simulink library "IO"  (R2025a)
settings: Solver=VariableStepAuto  StartTime=0.0  StopTime=10.0  RelTol=1e-3
values from neighbouring files (symbols this model uses):
  ADCBits = 12.0    [IO.sldd]
  Vref = 5.0    [IO.sldd]
undefined symbols (not defined in the file or in its folder): Bridge, dt, H, raptor_xcp_function
libraries: Raptor_lib x133, Utilities x20, Cooling x1
(part 6 of 6)

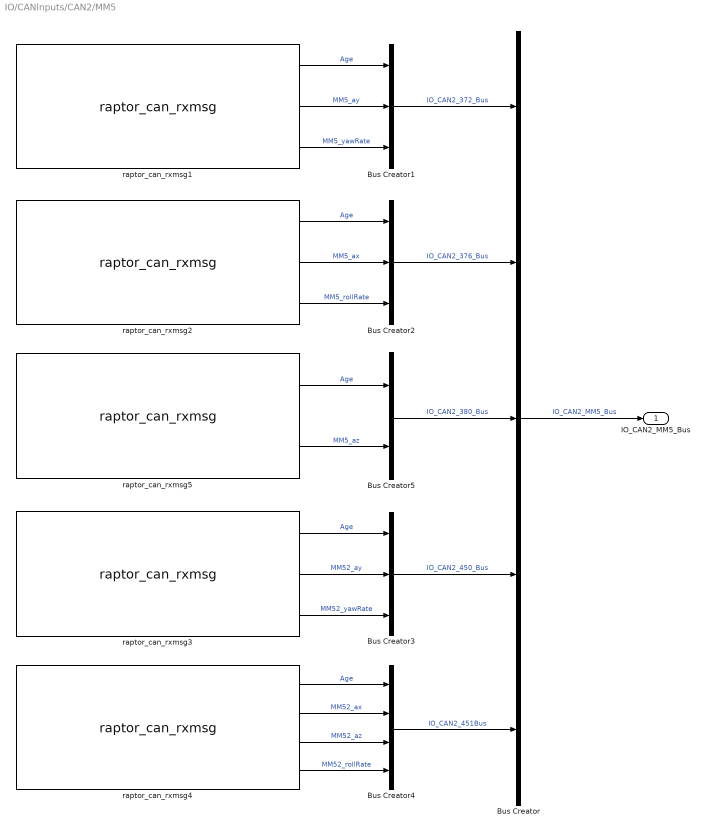
== system IO/CANInputs/CAN2/MM5 ==
  Bus Creator : BusCreator  Inputs=5
  Bus Creator1 : BusCreator  Inputs=3
  Bus Creator2 : BusCreator  Inputs=3
  Bus Creator3 : BusCreator  Inputs=3
  Bus Creator4 : BusCreator  Inputs=4
  Bus Creator5 : BusCreator  Inputs=2
  raptor_can_rxmsg1 : Raptor_lib/CAN/raptor_can_rxmsg  canDefinition=struct('dbcFile', 'SR26_CAN2.dbc','message', 'MM5_372','comment', '','signals', {{'MM5_ay','MM5_yawRate'}},'enabled', [ 1 1;],'scaled', [ 1 1;],'canBus', '''CAN2''','messageID', [ 372;],'idMask', [ 536870911;],'payloadMask', [],'payloadValue', [],'period', [ 0;],'mailbox', '''''','queueSize', [ 1;],'label', [ 0;],'ver', [ 2;],'showID', [ 0;],'showRaw', [ 0;],'showRawMsg', [ 0;],'useStartVals', [ 0;],'extendedId', [ 0;],'showAge', [ 1;],'useSimFunc', [ 0;],'sim_func_name', '''''','fill', [ 0;],'editID', [ 0;],'signalOrder', [ 1;],'signalAscDes', [ 1;],'msgLength', [ 8;])  canBus='CAN2'  mailbox=''  payloadMask=[]  payloadValue=[]  idMask=hex2dec('1FFFFFFF')  queueSize=1  showID=0  label=0  fill=0  id=372  showRaw=0  showAge=1  signalOrder=1  signalInfo={{struct('Name', 'MM5_ay','StartBit', [ 32;],'SignalSize', [ 16;],'ByteOrder', 'LittleEndian','ValueType', 'UNSIGNED','Class', 'uint16','Signed', [ 0;],'Factor', [ 0.0001274;],'Offset', [ -4.1746;],'Min', [ 0;],'Max', [ 0;],'Units', 'g','StartVal', [ 0;],'Comment', 'Acceleration Y Axis','Multiplexed', [ 0;],'Multiplexor', [ 0;],'MultiplexMode_Min', [],'MultiplexMode_Max', []),struct('Name', 'MM5_yawRate','StartBit', [ 0;],'SignalSize', [ 16;],'ByteOrder', 'LittleEndian','ValueType', 'UNSIGNED','Class', 'uint16','Signed', [ 0;],'Factor', [ 0.005;],'Offset', [ -163.9;],'Min', [ 0;],'Max', [ 0;],'Units', 'deg/sec','StartVal', [ 0;],'Comment', 'Yaw Rate','Multiplexed', [ 0;],'Multiplexor', [ 0;],'MultiplexMode_Min', [],'MultiplexMode_Max', [])}}  showRawMsg=0  useSimFunc=0  sim_func_name=''  useStartVals=0  extendedId=0
      settings: SourceProductName=Raptor
  raptor_can_rxmsg2 : Raptor_lib/CAN/raptor_can_rxmsg  canDefinition=struct('dbcFile', 'SR26_CAN2.dbc','message', 'MM5_376','comment', '','signals', {{'MM5_ax','MM5_rollRate'}},'enabled', [ 1 1;],'scaled', [ 1 1;],'canBus', '''CAN2''','messageID', [ 376;],'idMask', [ 536870911;],'payloadMask', [],'payloadValue', [],'period', [ 0;],'mailbox', '''''','queueSize', [ 1;],'label', [ 0;],'ver', [ 2;],'showID', [ 0;],'showRaw', [ 0;],'showRawMsg', [ 0;],'useStartVals', [ 0;],'extendedId', [ 0;],'showAge', [ 1;],'useSimFunc', [ 0;],'sim_func_name', '''''','fill', [ 0;],'editID', [ 0;],'signalOrder', [ 1;],'signalAscDes', [ 1;],'msgLength', [ 8;])  canBus='CAN2'  mailbox=''  payloadMask=[]  payloadValue=[]  idMask=hex2dec('1FFFFFFF')  queueSize=1  showID=0  label=0  fill=0  id=376  showRaw=0  showAge=1  signalOrder=1  signalInfo={{struct('Name', 'MM5_ax','StartBit', [ 32;],'SignalSize', [ 16;],'ByteOrder', 'LittleEndian','ValueType', 'UNSIGNED','Class', 'uint16','Signed', [ 0;],'Factor', [ -0.0001274;],'Offset', [ 4.1746;],'Min', [ 0;],'Max', [ 0;],'Units', 'g','StartVal', [ 0;],'Comment', 'Acceleration X Axis','Multiplexed', [ 0;],'Multiplexor', [ 0;],'MultiplexMode_Min', [],'MultiplexMode_Max', []),struct('Name', 'MM5_rollRate','StartBit', [ 0;],'SignalSize', [ 16;],'ByteOrder', 'LittleEndian','ValueType', 'UNSIGNED','Class', 'uint16','Signed', [ 0;],'Factor', [ -0.005;],'Offset', [ 163.9;],'Min', [ 0;],'Max', [ 0;],'Units', 'deg/sec','StartVal', [ 0;],'Comment', 'Roll Rate','Multiplexed', [ 0;],'Multiplexor', [ 0;],'MultiplexMode_Min', [],'MultiplexMode_Max', [])}}  showRawMsg=0  useSimFunc=0  sim_func_name=''  useStartVals=0  extendedId=0
      settings: SourceProductName=Raptor
  raptor_can_rxmsg3 : Raptor_lib/CAN/raptor_can_rxmsg  canDefinition=struct('dbcFile', 'SR26_CAN2.dbc','message', 'MM52_450','comment', '','signals', {{'MM52_ay','MM52_yawRate'}},'enabled', [ 1 1;],'scaled', [ 1 1;],'canBus', '''CAN2''','messageID', [ 450;],'idMask', [ 536870911;],'payloadMask', [],'payloadValue', [],'period', [ 0;],'mailbox', '''''','queueSize', [ 1;],'label', [ 0;],'ver', [ 2;],'showID', [ 0;],'showRaw', [ 0;],'showRawMsg', [ 0;],'useStartVals', [ 0;],'extendedId', [ 0;],'showAge', [ 1;],'useSimFunc', [ 0;],'sim_func_name', '''''','fill', [ 0;],'editID', [ 0;],'signalOrder', [ 1;],'signalAscDes', [ 1;],'msgLength', [ 8;])  canBus='CAN2'  mailbox=''  payloadMask=[]  payloadValue=[]  idMask=hex2dec('1FFFFFFF')  queueSize=1  showID=0  label=0  fill=0  id=450  showRaw=0  showAge=1  signalOrder=1  signalInfo={{struct('Name', 'MM52_ay','StartBit', [ 32;],'SignalSize', [ 16;],'ByteOrder', 'LittleEndian','ValueType', 'UNSIGNED','Class', 'uint16','Signed', [ 0;],'Factor', [ 0.0001274;],'Offset', [ -4.1746;],'Min', [ 0;],'Max', [ 0;],'Units', 'g','StartVal', [ 0;],'Comment', 'Acceleration Y Axis','Multiplexed', [ 0;],'Multiplexor', [ 0;],'MultiplexMode_Min', [],'MultiplexMode_Max', []),struct('Name', 'MM52_yawRate','StartBit', [ 0;],'SignalSize', [ 16;],'ByteOrder', 'LittleEndian','ValueType', 'UNSIGNED','Class', 'uint16','Signed', [ 0;],'Factor', [ 0.005;],'Offset', [ -163.9;],'Min', [ 0;],'Max', [ 0;],'Units', 'deg/sec','StartVal', [ 0;],'Comment', 'Yaw Rate','Multiplexed', [ 0;],'Multiplexor', [ 0;],'MultiplexMode_Min', [],'MultiplexMode_Max', [])}}  showRawMsg=0  useSimFunc=0  sim_func_name=''  useStartVals=0  extendedId=0
      settings: SourceProductName=Raptor
  raptor_can_rxmsg4 : Raptor_lib/CAN/raptor_can_rxmsg  canDefinition=struct('dbcFile', 'SR26_CAN2.dbc','message', 'MM52_451','comment', '','signals', {{'MM52_ax','MM52_az','MM52_rollRate'}},'enabled', [ 1 1 1;],'scaled', [ 1 1 1;],'canBus', '''CAN2''','messageID', [ 451;],'idMask', [ 536870911;],'payloadMask', [],'payloadValue', [],'period', [ 0;],'mailbox', '''''','queueSize', [ 1;],'label', [ 0;],'ver', [ 2;],'showID', [ 0;],'showRaw', [ 0;],'showRawMsg', [ 0;],'useStartVals', [ 0;],'extendedId', [ 0;],'showAge', [ 1;],'useSimFunc', [ 0;],'sim_func_name', '''''','fill', [ 0;],'editID', [ 0;],'signalOrder', [ 1;],'signalAscDes', [ 1;],'msgLength', [ 8;])  canBus='CAN2'  mailbox=''  payloadMask=[]  payloadValue=[]  idMask=hex2dec('1FFFFFFF')  queueSize=1  showID=0  label=0  fill=0  id=451  showRaw=0  showAge=1  signalOrder=1  signalInfo={{struct('Name', 'MM52_az','StartBit', [ 32;],'SignalSize', [ 16;],'ByteOrder', 'LittleEndian','ValueType', 'UNSIGNED','Class', 'uint16','Signed', [ 0;],'Factor', [ -0.0001274;],'Offset', [ 4.1746;],'Min', [ 0;],'Max', [ 0;],'Units', 'g','StartVal', [ 0;],'Comment', 'Acceleration Z Axis','Multiplexed', [ 0;],'Multiplexor', [ 0;],'MultiplexMode_Min', [],'MultiplexMode_Max', []),struct('Name', 'MM52_ax','StartBit', [ 16;],'SignalSize', [ 16;],'ByteOrder', 'LittleEndian','ValueType', 'UNSIGNED','Class', 'uint16','Signed', [ 0;],'Factor', [ -0.0001274;],'Offset', [ 4.1746;],'Min', [ 0;],'Max', [ 0;],'Units', 'g','StartVal', [ 0;],'Comment', 'Acceleration X Axis','Multiplexed', [ 0;],'Multiplexor', [ 0;],'MultiplexMode_Min', [],'MultiplexMode_Max', []),struct('Name', 'MM52_rollRate','StartBit', [ 0;],'SignalSize', [ 16;],'ByteOrder', 'LittleEndian','ValueType', 'UNSIGNED','Class', 'uint16','Signed', [ 0;],'Factor', [ -0.005;],'Offset', [ 163.9;],'Min', [ 0;],'Max', [ 0;],'Units', 'deg/sec','StartVal', [ 0;],'Comment', 'Roll Rate','Multiplexed', [ 0;],'Multiplexor', [ 0;],'MultiplexMode_Min', [],'MultiplexMode_Max', [])}}  showRawMsg=0  useSimFunc=0  sim_func_name=''  useStartVals=0  extendedId=0
      settings: SourceProductName=Raptor
  raptor_can_rxmsg5 : Raptor_lib/CAN/raptor_can_rxmsg  canDefinition=struct('dbcFile', 'SR26_CAN2.dbc','message', 'MM5_380','comment', '','signals', {{'MM5_az'}},'enabled', [ 1;],'scaled', [ 1;],'canBus', '''CAN2''','messageID', [ 380;],'idMask', [ 536870911;],'payloadMask', [],'payloadValue', [],'period', [ 0;],'mailbox', '''''','queueSize', [ 1;],'label', [ 0;],'ver', [ 2;],'showID', [ 0;],'showRaw', [ 0;],'showRawMsg', [ 0;],'useStartVals', [ 0;],'extendedId', [ 0;],'showAge', [ 1;],'useSimFunc', [ 0;],'sim_func_name', '''''','fill', [ 0;],'editID', [ 0;],'signalOrder', [ 1;],'signalAscDes', [ 1;],'msgLength', [ 8;])  canBus='CAN2'  mailbox=''  payloadMask=[]  payloadValue=[]  idMask=hex2dec('1FFFFFFF')  queueSize=1  showID=0  label=0  fill=0  id=380  showRaw=0  showAge=1  signalOrder=1  signalInfo={{struct('Name', 'MM5_az','StartBit', [ 32;],'SignalSize', [ 16;],'ByteOrder', 'LittleEndian','ValueType', 'UNSIGNED','Class', 'uint16','Signed', [ 0;],'Factor', [ -0.0001274;],'Offset', [ 4.1746;],'Min', [ 0;],'Max', [ 0;],'Units', 'g','StartVal', [ 0;],'Comment', 'Acceleration Z Axis','Multiplexed', [ 0;],'Multiplexor', [ 0;],'MultiplexMode_Min', [],'MultiplexMode_Max', [])}}  showRawMsg=0  useSimFunc=0  sim_func_name=''  useStartVals=0  extendedId=0
      settings: SourceProductName=Raptor
  IO_CAN2_MM5_Bus : Outport
  wires:
  raptor_can_rxmsg5/2 -> Bus Creator5/2  "MM5_az"
  raptor_can_rxmsg5/1 -> Bus Creator5/1  "Age"
  raptor_can_rxmsg2/3 -> Bus Creator2/3  "MM5_rollRate"
  raptor_can_rxmsg1/3 -> Bus Creator1/3  "MM5_yawRate"
  raptor_can_rxmsg4/4 -> Bus Creator4/4  "MM52_rollRate"
  Bus Creator5/1 -> Bus Creator/3  "IO_CAN2_380_Bus"
  Bus Creator3/1 -> Bus Creator/4  "IO_CAN2_450_Bus"
  raptor_can_rxmsg3/2 -> Bus Creator3/2  "MM52_ay"
  raptor_can_rxmsg3/1 -> Bus Creator3/1  "Age"
  Bus Creator4/1 -> Bus Creator/5  "IO_CAN2_451Bus"
  raptor_can_rxmsg3/3 -> Bus Creator3/3  "MM52_yawRate"
  raptor_can_rxmsg4/2 -> Bus Creator4/2  "MM52_ax"
  raptor_can_rxmsg4/3 -> Bus Creator4/3  "MM52_az"
  raptor_can_rxmsg4/1 -> Bus Creator4/1  "Age"
  raptor_can_rxmsg2/1 -> Bus Creator2/1  "Age"
  raptor_can_rxmsg2/2 -> Bus Creator2/2  "MM5_ax"
  Bus Creator/1 -> IO_CAN2_MM5_Bus/1  "IO_CAN2_MM5_Bus"
  Bus Creator2/1 -> Bus Creator/2  "IO_CAN2_376_Bus"
  raptor_can_rxmsg1/1 -> Bus Creator1/1  "Age"
  raptor_can_rxmsg1/2 -> Bus Creator1/2  "MM5_ay"
  Bus Creator1/1 -> Bus Creator/1  "IO_CAN2_372_Bus"
